simulink model "aircraft_pitch_response"  (R2024b)
settings: Solver=VariableStepAuto  StartTime=0.0  StopTime=10.0  RelTol=1e-3
settings Model: Creator=91964  LastModifiedBy=91964

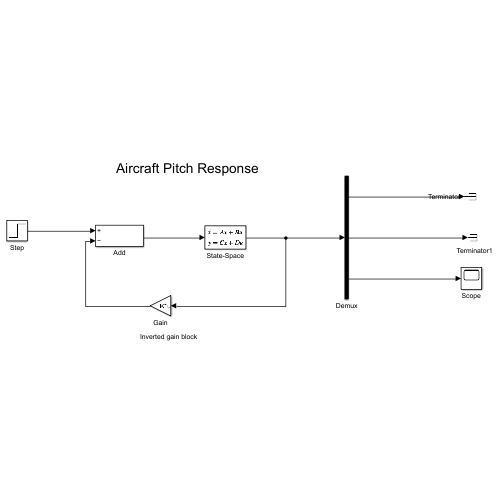
[thumbnail: Simulink's stored preview of the top-level diagram]
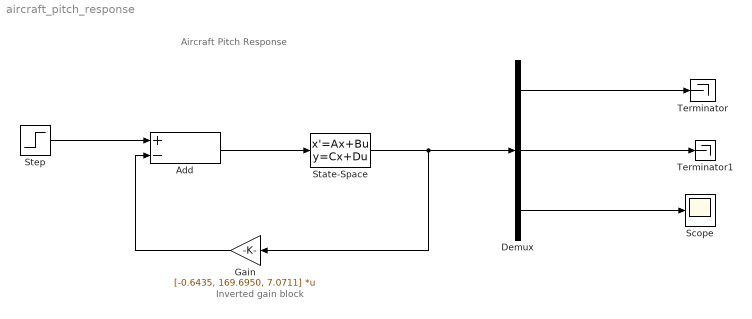
== system aircraft_pitch_response ==
  note: Inverted gain block
  note: Aircraft Pitch Response
  Add : Sum  Inputs=+-
  Demux : Demux  Outputs=3
  Gain : Gain  Gain=[-0.6435, 169.6950, 7.0711]  Multiplication=Matrix(K*u)
  Scope : Scope
  State-Space : StateSpace  A=[-0.313, 56.7, 0;-0.0139, -0.426, 0;0, 56.7, 0]  B=[0.232;0.0203;0]  C=eye(3)  D=[0;0;0]  InitialCondition=0  ContinuousStateAttributes={'Angle_of_attack','Pitch_rate','Pitch_Angle'}
  Step : Step  After=0.2  SampleTime=0
  Terminator : Terminator
  Terminator1 : Terminator
  wires:
  Demux/1 -> Terminator/1
  Demux/2 -> Terminator1/1
  Demux/3 -> Scope/1
  State-Space/1 -> Demux/1, Gain/1
  Gain/1 -> Add/2
  Step/1 -> Add/1
  Add/1 -> State-Space/1
